simulink model "gm_AMdemod2"  (R2021a)
settings: Solver=VariableStepAuto  StartTime=0.0  StopTime=10.0  RelTol=1e-3
libraries: hdlsllib x4, dspsrcs4 x3
settings Model: Creator=guido  LastModifiedBy=guido
settings OptimizationCC: BlockReduction=off  ConditionallyExecuteInputs=off  DefaultParameterBehavior=Inlined
settings DebuggingCC: AlgebraicLoopMsg=error  InheritedTsInSrcMsg=none
settings HardwareCC: ProdBitPerPointer=32  ProdBitPerSizeT=32  ProdBitPerPtrDiffT=32  ProdLargestAtomicFloat=None  ProdIntDivRoundTo=Undefined  ProdEndianess=Unspecified  ProdWordSize=32  ProdHWDeviceType=ASIC/FPGA->ASIC/FPGA  TargetBitPerPointer=64  TargetBitPerSizeT=64  TargetBitPerPtrDiffT=64  TargetLongLongMode=on  TargetIntDivRoundTo=Zero  TargetEndianess=LittleEndian  TargetWordSize=64  TargetHWDeviceType=Custom Processor->MATLAB Host Computer  ProdEqTarget=off

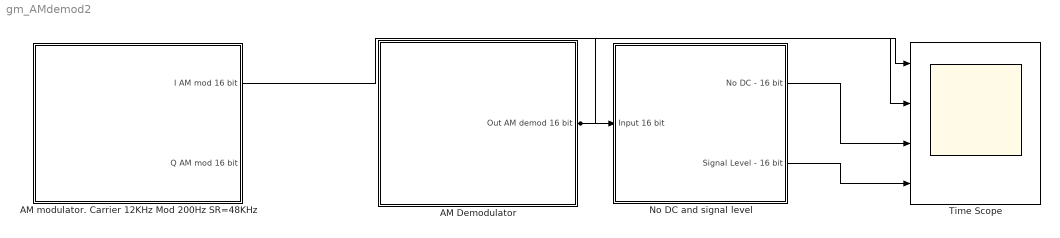
== system gm_AMdemod2 ==
  AM Demodulator : Subsystem
  "AM modulator. Carrier 12KHz Mod 200Hz SR=48KHz " : Subsystem
  No DC and signal level : Subsystem
  Time Scope : Scope  NumInputPorts=4
  wires:
  "AM modulator. Carrier 12KHz Mod 200Hz SR=48KHz "/1(I AM mod 16 bit) -> Time Scope/1
  AM Demodulator/1(Out AM demod 16 bit) -> No DC and signal level/1(Input 16 bit), Time Scope/2
  No DC and signal level/1(No DC - 16 bit) -> Time Scope/3
  No DC and signal level/2("Signal Level - 16 bit ") -> Time Scope/4

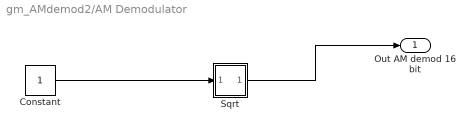
== system gm_AMdemod2/AM Demodulator ==
  Constant : Constant  OutDataTypeStr=int16  SampleTime=1
  Sqrt : Subsystem
  Out AM demod 16 bit : Outport  SampleTime=1
  wires:
  Constant/1 -> Sqrt/1(In1)
  Sqrt/1(Out1) -> Out AM demod 16 bit/1

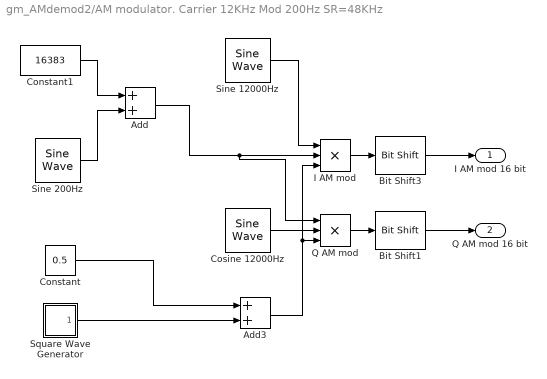
== system gm_AMdemod2/AM modulator. Carrier 12KHz Mod 200Hz SR=48KHz  ==
  Add : Sum  AccumDataTypeStr=int16  OutDataTypeStr=int16
  Add3 : Sum
  Bit Shift1 : hdlsllib/Logic and Bit Operations/Bit Shift  mode=Shift Right Arithmetic  N=16
  Bit Shift3 : hdlsllib/Logic and Bit Operations/Bit Shift  mode=Shift Right Arithmetic  N=16
  Constant : Constant  Value=0.5
  Constant1 : Constant  Value=16383  OutDataTypeStr=int16
  Cosine 12000Hz : dspsrcs4/Sine Wave  Amplitude=32767  Frequency=12000  Phase=pi/2  SampleMode=Discrete  OutComplex=Real  CompMethod=Table lookup  TableSize=Speed  SampleTime=1/48000  SamplesPerFrame=1  ResetState=Restart at time zero  OutputFrames=off  dataType=Fixed-point  wordLen=16  udDataType=sfix(16)  fracBitsMode=Best precision  numFracBits=0  OutDataTypeStr=fixdt(1,16)  LastOutDataTypeStr=fixdt(1,16)
  I AM mod : Product  Inputs=3  OutDataTypeStr=int32  SaturateOnIntegerOverflow=on
  Q AM mod : Product  Inputs=3  OutDataTypeStr=int32  SaturateOnIntegerOverflow=on
  Sine 12000Hz : dspsrcs4/Sine Wave  Amplitude=32767  Frequency=12000  Phase=0  SampleMode=Discrete  OutComplex=Real  CompMethod=Table lookup  TableSize=Speed  SampleTime=1/48000  SamplesPerFrame=1  ResetState=Restart at time zero  OutputFrames=off  dataType=Fixed-point  wordLen=16  udDataType=sfix(16)  fracBitsMode=Best precision  numFracBits=0  OutDataTypeStr=fixdt(1,16)  LastOutDataTypeStr=fixdt(1,16)
  Sine 200Hz : dspsrcs4/Sine Wave  Amplitude=16000  Frequency=800  Phase=0  SampleMode=Discrete  OutComplex=Real  CompMethod=Table lookup  TableSize=Speed  SampleTime=1/48000  SamplesPerFrame=1  ResetState=Restart at time zero  OutputFrames=off  dataType=Fixed-point  wordLen=16  udDataType=sfix(16)  fracBitsMode=Best precision  numFracBits=0  OutDataTypeStr=fixdt(1,16)  LastOutDataTypeStr=fixdt(1,16)
  Square Wave Generator : Subsystem  Tag=DecoupledSystem
  I AM mod 16 bit : Outport
  Q AM mod 16 bit : Outport  Port=2
  wires:
  Bit Shift1/1 -> Q AM mod 16 bit/1
  Bit Shift3/1 -> I AM mod 16 bit/1
  Q AM mod/1 -> Bit Shift1/1
  I AM mod/1 -> Bit Shift3/1
  Constant1/1 -> Add/1
  Square Wave Generator/1(Out1) -> Add3/2
  Sine 200Hz/1 -> Add/2
  Constant/1 -> Add3/1
  Cosine 12000Hz/1 -> Q AM mod/2
  Add/1 -> I AM mod/2, Q AM mod/1
  Sine 12000Hz/1 -> I AM mod/1
  Add3/1 -> Q AM mod/3, I AM mod/3

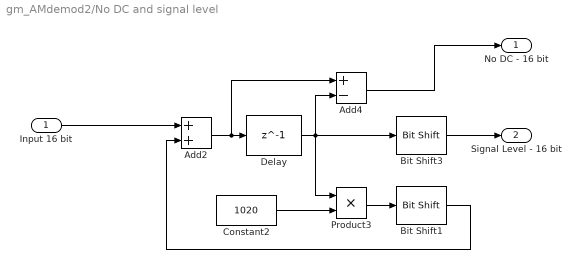
== system gm_AMdemod2/No DC and signal level ==
  Input 16 bit : Inport
  Add2 : Sum  AccumDataTypeStr=int64  OutDataTypeStr=int64
  Add4 : Sum  Inputs=+-  AccumDataTypeStr=int32  OutDataTypeStr=int16
  Bit Shift1 : hdlsllib/Logic and Bit Operations/Bit Shift  mode=Shift Right Arithmetic  N=10
  Bit Shift3 : hdlsllib/Logic and Bit Operations/Bit Shift  mode=Shift Right Arithmetic  N=9
  Constant2 : Constant  Value=1020  OutDataTypeStr=int32
  Delay : Delay  DelayLength=1  InitialCondition=1  UseCircularBuffer=on
  Product3 : Product  OutDataTypeStr=int64
  No DC - 16 bit : Outport
  "Signal Level - 16 bit " : Outport  Port=2
  wires:
  Add4/1 -> No DC - 16 bit/1
  Product3/1 -> Bit Shift1/1
  Bit Shift3/1 -> "Signal Level - 16 bit "/1
  Bit Shift1/1 -> Add2/2
  Add2/1 -> Delay/1, Add4/1
  Input 16 bit/1 -> Add2/1
  Constant2/1 -> Product3/2
  Delay/1 -> Add4/2, Bit Shift3/1, Product3/1

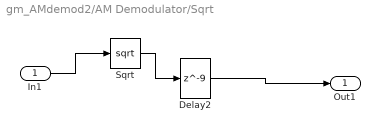
== system gm_AMdemod2/AM Demodulator/Sqrt ==
  In1 : Inport
  Delay2 : Delay  DelayLength=9
  Sqrt : Sqrt  SaturateOnIntegerOverflow=on  OutDataTypeStr=Inherit: Inherit via internal rule
  Out1 : Outport
  wires:
  In1/1 -> Sqrt/1
  Sqrt/1 -> Delay2/1
  Delay2/1 -> Out1/1

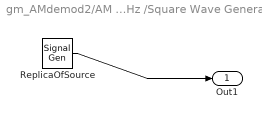
== system gm_AMdemod2/AM modulator. Carrier 12KHz Mod 200Hz SR=48KHz /Square Wave Generator ==
  ReplicaOfSource : SignalGenerator  WaveForm=square  Amplitude=0.5  Frequency=0.5
  Out1 : Outport  LockScale=on
  wires:
  ReplicaOfSource/1 -> Out1/1
